simulink library "walkingRobotUtils"  (R2023a)
settings: Solver=VariableStepAuto  StartTime=0.0  StopTime=10.0  RelTol=1e-3
values from neighbouring files (symbols this model uses):
  ankle_servo_kd = 8    [robotParametersCtrl_mydiem_block_zmp.m]    (also in robotParametersCtrl_quad_modify_mydiem.m; robotParametersCtrl_quad_modify_mydiem_reaction.m)
  ankle_servo_ki = 4    [robotParametersCtrl_mydiem_block_zmp.m]    (also in robotParametersCtrl_quad_modify_mydiem.m; robotParametersCtrl_quad_modify_mydiem_reaction.m)
  ankle_servo_kp = 20    [robotParametersCtrl_mydiem_block_zmp.m]    (also in robotParametersCtrl_quad_modify_mydiem.m; robotParametersCtrl_quad_modify_mydiem_reaction.m)
  deriv_filter_coeff = 100    [robotParametersCtrl_mydiem_block_zmp.m]    (also in robotParametersCtrl_quad_modify_mydiem.m; robotParametersCtrl_quad_modify_mydiem_reaction.m)
  foot_x = 9    [robotParametersCtrl_mydiem_block_zmp.m]    (also in robotParametersCtrl_quad_modify_mydiem.m; robotParametersCtrl_quad_modify_mydiem_reaction.m)
  foot_y = 5    [robotParametersCtrl_mydiem_block_zmp.m]    (also in robotParametersCtrl_quad_modify_mydiem.m; robotParametersCtrl_quad_modify_mydiem_reaction.m)
  foot_z = 1.5    [robotParametersCtrl_mydiem_block_zmp.m]    (also in robotParametersCtrl_quad_modify_mydiem.m; robotParametersCtrl_quad_modify_mydiem_reaction.m)
  height_plane = 0.025    [robotParametersCtrl_mydiem_block_zmp.m]    (also in robotParametersCtrl_quad_modify_mydiem.m; robotParametersCtrl_quad_modify_mydiem_reaction.m)
  hip_servo_kd = 20    [robotParametersCtrl_mydiem_block_zmp.m]    (also in robotParametersCtrl_quad_modify_mydiem.m; robotParametersCtrl_quad_modify_mydiem_reaction.m)
  hip_servo_ki = 10    [robotParametersCtrl_mydiem_block_zmp.m]    (also in robotParametersCtrl_quad_modify_mydiem.m; robotParametersCtrl_quad_modify_mydiem_reaction.m)
  hip_servo_kp = 60    [robotParametersCtrl_mydiem_block_zmp.m]    (also in robotParametersCtrl_quad_modify_mydiem.m; robotParametersCtrl_quad_modify_mydiem_reaction.m)
  init_angs_L = init_angs_R    [robotParametersCtrl_mydiem_block_zmp.m]    (also in robotParametersCtrl_quad_modify_mydiem.m; robotParametersCtrl_quad_modify_mydiem_reaction.m)
  init_angs_R = [0 -sum(init_angs) init_angs(2) 0 init_angs(1)]    [robotParametersCtrl_mydiem_block_zmp.m]    (also in robotParametersCtrl_quad_modify_mydiem.m; robotParametersCtrl_quad_modify_mydiem_reaction.m)
  init_height = h +                torso_z/2 + torso_offset_z + height_plane/2    (= 39.5125)    [robotParametersCtrl_mydiem_block_zmp.m]    (also in robotParametersCtrl_quad_modify_mydiem.m; robotParametersCtrl_quad_modify_mydiem_reaction.m)
  joint_damping = 1    [robotParametersCtrl_mydiem_block_zmp.m]    (also in robotParametersCtrl_quad_modify_mydiem.m; robotParametersCtrl_quad_modify_mydiem_reaction.m)
  knee_servo_kd = 10    [robotParametersCtrl_mydiem_block_zmp.m]    (also in robotParametersCtrl_quad_modify_mydiem.m; robotParametersCtrl_quad_modify_mydiem_reaction.m)
  knee_servo_ki = 5    [robotParametersCtrl_mydiem_block_zmp.m]    (also in robotParametersCtrl_quad_modify_mydiem.m; robotParametersCtrl_quad_modify_mydiem_reaction.m)
  knee_servo_kp = 60    [robotParametersCtrl_mydiem_block_zmp.m]    (also in robotParametersCtrl_quad_modify_mydiem.m; robotParametersCtrl_quad_modify_mydiem_reaction.m)
  lower_leg_length = 20    [robotParametersCtrl_mydiem_block_zmp.m]    (also in robotParametersCtrl_quad_modify_mydiem.m; robotParametersCtrl_quad_modify_mydiem_reaction.m)
  max_torque = 20    [robotParametersCtrl_mydiem_block_zmp.m]    (also in robotParametersCtrl_quad_modify_mydiem.m; robotParametersCtrl_quad_modify_mydiem_reaction.m)
  motion_time_constant = 0.01    [robotParametersCtrl_mydiem_block_zmp.m]    (also in robotParametersCtrl_quad_modify_mydiem.m; robotParametersCtrl_quad_modify_mydiem_reaction.m)
  motor_constant = 0.02    [robotParametersCtrl_mydiem_block_zmp.m]    (also in robotParametersCtrl_quad_modify_mydiem.m; robotParametersCtrl_quad_modify_mydiem_reaction.m)
  motor_inertia = 0    [robotParametersCtrl_mydiem_block_zmp.m]    (also in robotParametersCtrl_quad_modify_mydiem.m; robotParametersCtrl_quad_modify_mydiem_reaction.m)
  motor_voltage = 24    [robotParametersCtrl_mydiem_block_zmp.m]    (also in robotParametersCtrl_quad_modify_mydiem.m; robotParametersCtrl_quad_modify_mydiem_reaction.m)
  plane_x = 25    [robotParametersCtrl_mydiem_block_zmp.m]    (also in robotParametersCtrl_quad_modify_mydiem.m; robotParametersCtrl_quad_modify_mydiem_reaction.m)
  plane_y = 3    [robotParametersCtrl_mydiem_block_zmp.m]    (also in robotParametersCtrl_quad_modify_mydiem.m; robotParametersCtrl_quad_modify_mydiem_reaction.m)
  torso_offset_x = 17    [robotParametersCtrl_mydiem_block_zmp.m]    (also in robotParametersCtrl_quad_modify_mydiem.m; robotParametersCtrl_quad_modify_mydiem_reaction.m)
  torso_offset_z = 0    [robotParametersCtrl_mydiem_block_zmp.m]    (also in robotParametersCtrl_quad_modify_mydiem.m; robotParametersCtrl_quad_modify_mydiem_reaction.m)
  torso_x = 40    [robotParametersCtrl_mydiem_block_zmp.m]    (also in robotParametersCtrl_quad_modify_mydiem.m; robotParametersCtrl_quad_modify_mydiem_reaction.m)
  torso_y = 20    [robotParametersCtrl_mydiem_block_zmp.m]    (also in robotParametersCtrl_quad_modify_mydiem.m; robotParametersCtrl_quad_modify_mydiem_reaction.m)
  torso_z = 15    [robotParametersCtrl_mydiem_block_zmp.m]    (also in robotParametersCtrl_quad_modify_mydiem.m; robotParametersCtrl_quad_modify_mydiem_reaction.m)
  upper_leg_length = 20    [robotParametersCtrl_mydiem_block_zmp.m]    (also in robotParametersCtrl_quad_modify_mydiem.m; robotParametersCtrl_quad_modify_mydiem_reaction.m)
undefined symbols (not defined in the file or in its folder): leg_width, plane_z, torso_height, torso_length, torso_offset_height, torso_offset_length, torso_width, X, Y, Z
libraries: sm_lib x110, nesl_utility x49, simulink x33, simulink_extras x32, $bdroot x28, fl_lib x7, ee_lib x3, Multibody_Multiphysics_Lib x1
(part 4 of 6)

== system walkingRobotUtils/Walking Robot (Control Design)/World and Ground ==
  Mechanism Configuration : sm_lib/Utilities/Mechanism Configuration  UniformGravity=Constant  GravityVector=[0 0 -9.80665]  GravityVectorUnits=m/s^2  LinearizationDelta=0.001  JointModeTransitionNonlinearIterations=2
  Plane Offset : sm_lib/Frames and Transforms/Rigid Transform  TranslationMethod=StandardAxis  TranslationStandardOffset=height_plane/2  TranslationStandardOffsetUnits=m  TranslationStandardAxis=-Z  TranslationCartesianOffset=[0 0 0]  TranslationCartesianOffsetUnits=m  TranslationROffset=0  TranslationROffsetUnits=m  TranslationZOffset=0  TranslationZOffsetUnits=m  TranslationThetaOffset=0  TranslationThetaOffsetUnits=deg  RotationMethod=None  RotationAngleUnits=deg  RotationStandardAxis=+Z  RotationAngle=0.0  RotationArbitraryAxis=[0 0 1]  FollAlignAxisA=+X  BaseAlignAxisA=+Y  FollAlignAxisB=+Y  BaseAlignAxisB=+Z  RotationSequenceAxes=FollowerAxes  RotationSequence=XYX  RotationSequenceAngles=[0 0 0]  RotationSequenceAnglesUnits=deg  RotationMatrix=[1 0 0; 0 1 0; 0 0 1]  Quaternion=[1 0 0 0]
  Solver Configuration : nesl_utility/Solver Configuration  PhysicalDomain=network_engine_domain  SubClassName=solver  LeftPortType=input  RightPortType=generic  Tones=[]  Harmonics=[]  SimulateNoise=off  Profile=off  UseLocalSampling=off  EnableSwitchedLinearOptims=on  FrequencyDomain=off  UseCCode=off  RelTol=0.001  AbsTol=1e-06  MinStep=1e-09  ToWorkspace=off  RevertToSquareIcSolve=off  NumHomotopyIterations=100  PhasorMode=off  PhasorModeNumHarmonics=1  ConsistencySolver=NEWTON_FTOL  IndexReductionMethod=DerivativeReplacement  DoDC=off  ResidualTolerance=1e-09  ConsistencyTolSource=GLOBAL  ConsistencyAbsTol=0.001  ConsistencyRelTol=0.001  ConsistencyTolFactor=0.001  UseLocalSolver=off  LocalSolverChoice=NE_TRAPEZOIDAL_ADVANCER  ResolveIndetEquations=on  FunctionEvalNumThread=1  LocalSolverSampleTime=0.01  DoFixedCost=off  MaxNonlinIter=3  MaxModeIter=2  ComputeImpulses=off  ImpulseIterations=2  LinearAlgebra=Sparse  LinearAlgebraNumThread=0  EquationFormulation=NE_TIME_EF  DelaysMemoryBudget=1024  AutomaticFiltering=on  FilteringTimeConstant=0.001  PartitionStorageMethod=AS_NEEDED  PartitionMemoryBudget=1024  PartitionMethod=FAST
  World Frame1 : sm_lib/Frames and Transforms/World Frame
  World Plane : sm_lib/Body Elements/Brick Solid  GraphicAmbientColor=[0.15 0.15 0.15 1.0]  BasedOnType=Density  BrickDimensions="[plane_x plane_y  height_plane]"  BrickDimensionsUnits=m  CenterOfMass=[0 0 0]  CenterOfMassUnits=m  GraphicDiffuseColor=[1.0 1.0 0.8]  Density=density  DensityUnits=kg/(m^3)  DoExposeReferenceFrame=on  GraphicEmissiveColor=[0.0 0.0 0.0 1.0]  ExportEntireGeometry=on  SerializedFrames=<Frames/>  MarkerShape=Sphere  MarkerSize=10  GraphicType=FromGeometry  InertiaType=CalculateFromGeometry  Mass=1  MassUnits=kg  MomentsOfInertia=[1 1 1]  MomentsOfInertiaUnits=kg*m^2  GraphicOpacity=0.5  ProductsOfInertia=[0 0 0]  ProductsOfInertiaUnits=kg*m^2  GraphicShininess=75  GraphicSpecularColor=[0.5 0.5 0.5 1.0]  GraphicVisPropType=SimpleVisualProperties
  W : PMIOPort  Side=Left
  G : PMIOPort  Port=2  Side=Right
  connections:
  World Frame1/RConn1 -- W/RConn1 -- Mechanism Configuration/RConn1 -- Plane Offset/LConn1 -- Solver Configuration/RConn1
  World Plane/RConn1 -- Plane Offset/RConn1
  G/RConn1 -- World Plane/LConn1

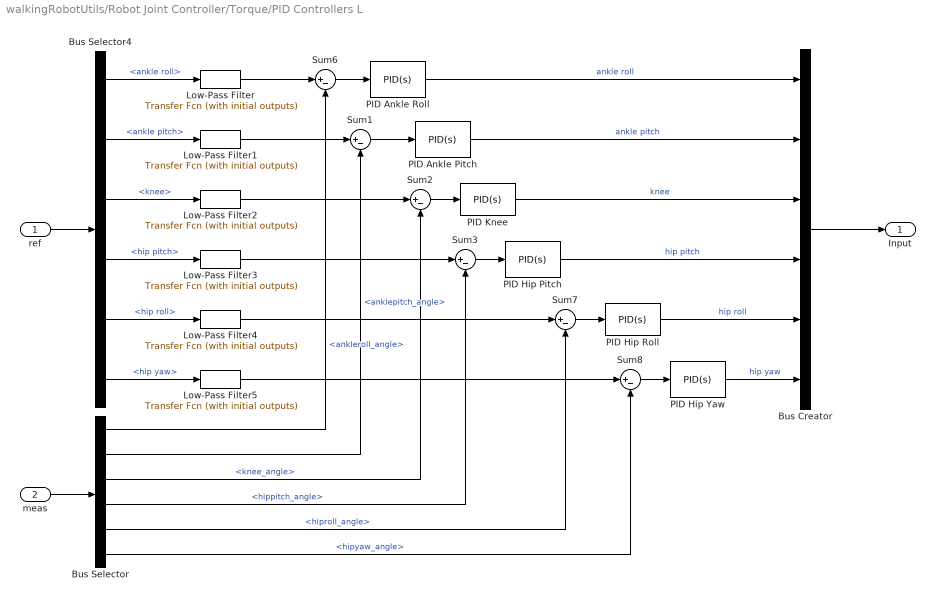
== system walkingRobotUtils/Robot Joint Controller/Torque/PID Controllers L ==
  ref : Inport
  meas : Inport  Port=2
  Bus Creator : BusCreator  Inputs=6
  Bus Selector : BusSelector  OutputSignals=ankleroll_angle,anklepitch_angle,knee_angle,hippitch_angle,hiproll_angle,hipyaw_angle
  Bus Selector4 : BusSelector  OutputSignals=ankle roll,ankle pitch,knee,hip pitch,hip roll,hip yaw
  Low-Pass Filter : simulink_extras/Additional Linear/Transfer Fcn (with initial outputs)  N=[(1/motion_time_constant)^2]  D=[1 2/motion_time_constant (1/motion_time_constant)^2]  Y0=init_angs_L(6)  U0=init_angs_L(6)
  Low-Pass Filter1 : simulink_extras/Additional Linear/Transfer Fcn (with initial outputs)  N=[(1/motion_time_constant)^2]  D=[1 2/motion_time_constant (1/motion_time_constant)^2]  Y0=init_angs_L(5)  U0=init_angs_L(5)
  Low-Pass Filter2 : simulink_extras/Additional Linear/Transfer Fcn (with initial outputs)  N=[(1/motion_time_constant)^2]  D=[1 2/motion_time_constant (1/motion_time_constant)^2]  Y0=init_angs_L(4)  U0=init_angs_L(4)
  Low-Pass Filter3 : simulink_extras/Additional Linear/Transfer Fcn (with initial outputs)  N=[(1/motion_time_constant)^2]  D=[1 2/motion_time_constant (1/motion_time_constant)^2]  Y0=init_angs_L(3)  U0=init_angs_L(3)
  Low-Pass Filter4 : simulink_extras/Additional Linear/Transfer Fcn (with initial outputs)  N=[(1/motion_time_constant)^2]  D=[1 2/motion_time_constant (1/motion_time_constant)^2]  Y0=init_angs_L(2)  U0=init_angs_L(2)
  Low-Pass Filter5 : simulink_extras/Additional Linear/Transfer Fcn (with initial outputs)  N=[(1/motion_time_constant)^2]  D=[1 2/motion_time_constant (1/motion_time_constant)^2]  Y0=init_angs_L(1)  U0=init_angs_L(1)
  PID Ankle Pitch : simulink/Continuous/PID Controller  Controller=PID  Form=Parallel  TimeDomain=Continuous-time  SampleTime=-1  IntegratorMethod=Forward Euler  FilterMethod=Forward Euler  ControllerParametersSource=internal  P=ankle_servo_kp  I=ankle_servo_ki  D=ankle_servo_kd  UseFilter=on  N=deriv_filter_coeff  TunerSelectOption=Transfer Function Based (PID Tuner App)  ZeroCross=off  InitialConditionSource=internal  InitialConditionForIntegrator=0  InitialConditionForFilter=0  DifferentiatorICPrevScaledInput=0  ExternalReset=none  TrackingMode=off  Kt=1  LimitOutput=on  UpperSaturationLimit=max_torque  LowerSaturationLimit=-max_torque  LinearizeAsGain=on  AntiWindupMode=clamping  Kb=1  POutMin=[]  POutMax=[]  IOutMin=[]  IOutMax=[]  DOutMin=[]  DOutMax=[]  NOutMin=[]  NOutMax=[]  SumOutMin=[]  SumOutMax=[]  SaturationOutMin=[]  SaturationOutMax=[]  PParamMin=[]  PParamMax=[]  IParamMin=[]  IParamMax=[]  DParamMin=[]  DParamMax=[]  NParamMin=[]  NParamMax=[]  KbParamMin=[]  KbParamMax=[]  KtParamMin=[]  KtParamMax=[]  KbOutMin=[]  KbOutMax=[]  KtOutMin=[]  KtOutMax=[]  IntegratorOutMin=[]  IntegratorOutMax=[]  FilterOutMin=[]  FilterOutMax=[]  SumI1OutMin=[]  SumI1OutMax=[]  SumI2OutMin=[]  SumI2OutMax=[]  SumI3OutMin=[]  SumI3OutMax=[]  SumI4OutMin=[]  SumI4OutMax=[]  SumDOutMin=[]  SumDOutMax=[]  DifferentiatorOutMin=[]  DifferentiatorOutMax=[]  FilterDiffOutCoefMin=[]  FilterDiffOutCoefMax=[]  ReciprocalOutMin=[]  ReciprocalOutMax=[]  SumDenOutMin=[]  SumDenOutMax=[]  SumNumOutMin=[]  SumNumOutMax=[]  DivideOutMin=[]  DivideOutMax=[]  IntegratorContinuousStateAttributes=''  IntegratorStateMustResolveToSignalObject=off  IntegratorRTWStateStorageClass=Auto  FilterContinuousStateAttributes=''  FilterStateMustResolveToSignalObject=off  FilterRTWStateStorageClass=Auto  ParallelPVariant=InternalParameters  IdealPVariant=Disabled  IVariant=InternalParameters  DVariant=InternalParameters  IntegratorVariant=Continuous  SatVariant=Enabled  AWVariant=ContClampingParallel  PCopyVariant=Disabled  TRVariant=Disabled  FdbkBlocksVariant=Forward  IdealPFdbkVariant=Disabled  SatFdbkVariant=Disabled  DerivativeFilterVariant=ContFilter  NVariant=InternalParameters  NCopyVariant=Disabled  FilterICVariant=InternalICsFilter  IntegratorICVariant=InternalICs  ExternalResetVariant=Disabled  TRSumVariant=Passthrough  SumFdbkVariant=Disabled  SumVariant=Sum_PID
  PID Ankle Roll : simulink/Continuous/PID Controller  Controller=PID  Form=Parallel  TimeDomain=Continuous-time  SampleTime=-1  IntegratorMethod=Forward Euler  FilterMethod=Forward Euler  ControllerParametersSource=internal  P=ankle_servo_kp  I=ankle_servo_ki  D=ankle_servo_kd  UseFilter=on  N=deriv_filter_coeff  TunerSelectOption=Transfer Function Based (PID Tuner App)  ZeroCross=off  InitialConditionSource=internal  InitialConditionForIntegrator=0  InitialConditionForFilter=0  DifferentiatorICPrevScaledInput=0  ExternalReset=none  TrackingMode=off  Kt=1  LimitOutput=on  UpperSaturationLimit=max_torque  LowerSaturationLimit=-max_torque  LinearizeAsGain=on  AntiWindupMode=clamping  Kb=1  POutMin=[]  POutMax=[]  IOutMin=[]  IOutMax=[]  DOutMin=[]  DOutMax=[]  NOutMin=[]  NOutMax=[]  SumOutMin=[]  SumOutMax=[]  SaturationOutMin=[]  SaturationOutMax=[]  PParamMin=[]  PParamMax=[]  IParamMin=[]  IParamMax=[]  DParamMin=[]  DParamMax=[]  NParamMin=[]  NParamMax=[]  KbParamMin=[]  KbParamMax=[]  KtParamMin=[]  KtParamMax=[]  KbOutMin=[]  KbOutMax=[]  KtOutMin=[]  KtOutMax=[]  IntegratorOutMin=[]  IntegratorOutMax=[]  FilterOutMin=[]  FilterOutMax=[]  SumI1OutMin=[]  SumI1OutMax=[]  SumI2OutMin=[]  SumI2OutMax=[]  SumI3OutMin=[]  SumI3OutMax=[]  SumI4OutMin=[]  SumI4OutMax=[]  SumDOutMin=[]  SumDOutMax=[]  DifferentiatorOutMin=[]  DifferentiatorOutMax=[]  FilterDiffOutCoefMin=[]  FilterDiffOutCoefMax=[]  ReciprocalOutMin=[]  ReciprocalOutMax=[]  SumDenOutMin=[]  SumDenOutMax=[]  SumNumOutMin=[]  SumNumOutMax=[]  DivideOutMin=[]  DivideOutMax=[]  IntegratorContinuousStateAttributes=''  IntegratorStateMustResolveToSignalObject=off  IntegratorRTWStateStorageClass=Auto  FilterContinuousStateAttributes=''  FilterStateMustResolveToSignalObject=off  FilterRTWStateStorageClass=Auto  ParallelPVariant=InternalParameters  IdealPVariant=Disabled  IVariant=InternalParameters  DVariant=InternalParameters  IntegratorVariant=Continuous  SatVariant=Enabled  AWVariant=ContClampingParallel  PCopyVariant=Disabled  TRVariant=Disabled  FdbkBlocksVariant=Forward  IdealPFdbkVariant=Disabled  SatFdbkVariant=Disabled  DerivativeFilterVariant=ContFilter  NVariant=InternalParameters  NCopyVariant=Disabled  FilterICVariant=InternalICsFilter  IntegratorICVariant=InternalICs  ExternalResetVariant=Disabled  TRSumVariant=Passthrough  SumFdbkVariant=Disabled  SumVariant=Sum_PID
  PID Hip Pitch : simulink/Continuous/PID Controller  Controller=PID  Form=Parallel  TimeDomain=Continuous-time  SampleTime=-1  IntegratorMethod=Forward Euler  FilterMethod=Forward Euler  ControllerParametersSource=internal  P=hip_servo_kp  I=hip_servo_ki  D=hip_servo_kd  UseFilter=on  N=deriv_filter_coeff  TunerSelectOption=Transfer Function Based (PID Tuner App)  ZeroCross=off  InitialConditionSource=internal  InitialConditionForIntegrator=0  InitialConditionForFilter=0  DifferentiatorICPrevScaledInput=0  ExternalReset=none  TrackingMode=off  Kt=1  LimitOutput=on  UpperSaturationLimit=max_torque  LowerSaturationLimit=-max_torque  LinearizeAsGain=on  AntiWindupMode=clamping  Kb=1  POutMin=[]  POutMax=[]  IOutMin=[]  IOutMax=[]  DOutMin=[]  DOutMax=[]  NOutMin=[]  NOutMax=[]  SumOutMin=[]  SumOutMax=[]  SaturationOutMin=[]  SaturationOutMax=[]  PParamMin=[]  PParamMax=[]  IParamMin=[]  IParamMax=[]  DParamMin=[]  DParamMax=[]  NParamMin=[]  NParamMax=[]  KbParamMin=[]  KbParamMax=[]  KtParamMin=[]  KtParamMax=[]  KbOutMin=[]  KbOutMax=[]  KtOutMin=[]  KtOutMax=[]  IntegratorOutMin=[]  IntegratorOutMax=[]  FilterOutMin=[]  FilterOutMax=[]  SumI1OutMin=[]  SumI1OutMax=[]  SumI2OutMin=[]  SumI2OutMax=[]  SumI3OutMin=[]  SumI3OutMax=[]  SumI4OutMin=[]  SumI4OutMax=[]  SumDOutMin=[]  SumDOutMax=[]  DifferentiatorOutMin=[]  DifferentiatorOutMax=[]  FilterDiffOutCoefMin=[]  FilterDiffOutCoefMax=[]  ReciprocalOutMin=[]  ReciprocalOutMax=[]  SumDenOutMin=[]  SumDenOutMax=[]  SumNumOutMin=[]  SumNumOutMax=[]  DivideOutMin=[]  DivideOutMax=[]  IntegratorContinuousStateAttributes=''  IntegratorStateMustResolveToSignalObject=off  IntegratorRTWStateStorageClass=Auto  FilterContinuousStateAttributes=''  FilterStateMustResolveToSignalObject=off  FilterRTWStateStorageClass=Auto  ParallelPVariant=InternalParameters  IdealPVariant=Disabled  IVariant=InternalParameters  DVariant=InternalParameters  IntegratorVariant=Continuous  SatVariant=Enabled  AWVariant=ContClampingParallel  PCopyVariant=Disabled  TRVariant=Disabled  FdbkBlocksVariant=Forward  IdealPFdbkVariant=Disabled  SatFdbkVariant=Disabled  DerivativeFilterVariant=ContFilter  NVariant=InternalParameters  NCopyVariant=Disabled  FilterICVariant=InternalICsFilter  IntegratorICVariant=InternalICs  ExternalResetVariant=Disabled  TRSumVariant=Passthrough  SumFdbkVariant=Disabled  SumVariant=Sum_PID
  PID Hip Roll : simulink/Continuous/PID Controller  Controller=PID  Form=Parallel  TimeDomain=Continuous-time  SampleTime=-1  IntegratorMethod=Forward Euler  FilterMethod=Forward Euler  ControllerParametersSource=internal  P=hip_servo_kp  I=hip_servo_ki  D=hip_servo_kd  UseFilter=on  N=deriv_filter_coeff  TunerSelectOption=Transfer Function Based (PID Tuner App)  ZeroCross=off  InitialConditionSource=internal  InitialConditionForIntegrator=0  InitialConditionForFilter=0  DifferentiatorICPrevScaledInput=0  ExternalReset=none  TrackingMode=off  Kt=1  LimitOutput=on  UpperSaturationLimit=max_torque  LowerSaturationLimit=-max_torque  LinearizeAsGain=on  AntiWindupMode=clamping  Kb=1  POutMin=[]  POutMax=[]  IOutMin=[]  IOutMax=[]  DOutMin=[]  DOutMax=[]  NOutMin=[]  NOutMax=[]  SumOutMin=[]  SumOutMax=[]  SaturationOutMin=[]  SaturationOutMax=[]  PParamMin=[]  PParamMax=[]  IParamMin=[]  IParamMax=[]  DParamMin=[]  DParamMax=[]  NParamMin=[]  NParamMax=[]  KbParamMin=[]  KbParamMax=[]  KtParamMin=[]  KtParamMax=[]  KbOutMin=[]  KbOutMax=[]  KtOutMin=[]  KtOutMax=[]  IntegratorOutMin=[]  IntegratorOutMax=[]  FilterOutMin=[]  FilterOutMax=[]  SumI1OutMin=[]  SumI1OutMax=[]  SumI2OutMin=[]  SumI2OutMax=[]  SumI3OutMin=[]  SumI3OutMax=[]  SumI4OutMin=[]  SumI4OutMax=[]  SumDOutMin=[]  SumDOutMax=[]  DifferentiatorOutMin=[]  DifferentiatorOutMax=[]  FilterDiffOutCoefMin=[]  FilterDiffOutCoefMax=[]  ReciprocalOutMin=[]  ReciprocalOutMax=[]  SumDenOutMin=[]  SumDenOutMax=[]  SumNumOutMin=[]  SumNumOutMax=[]  DivideOutMin=[]  DivideOutMax=[]  IntegratorContinuousStateAttributes=''  IntegratorStateMustResolveToSignalObject=off  IntegratorRTWStateStorageClass=Auto  FilterContinuousStateAttributes=''  FilterStateMustResolveToSignalObject=off  FilterRTWStateStorageClass=Auto  ParallelPVariant=InternalParameters  IdealPVariant=Disabled  IVariant=InternalParameters  DVariant=InternalParameters  IntegratorVariant=Continuous  SatVariant=Enabled  AWVariant=ContClampingParallel  PCopyVariant=Disabled  TRVariant=Disabled  FdbkBlocksVariant=Forward  IdealPFdbkVariant=Disabled  SatFdbkVariant=Disabled  DerivativeFilterVariant=ContFilter  NVariant=InternalParameters  NCopyVariant=Disabled  FilterICVariant=InternalICsFilter  IntegratorICVariant=InternalICs  ExternalResetVariant=Disabled  TRSumVariant=Passthrough  SumFdbkVariant=Disabled  SumVariant=Sum_PID
  PID Hip Yaw : simulink/Continuous/PID Controller  Controller=PID  Form=Parallel  TimeDomain=Continuous-time  SampleTime=-1  IntegratorMethod=Forward Euler  FilterMethod=Forward Euler  ControllerParametersSource=internal  P=hip_servo_kp  I=hip_servo_ki  D=hip_servo_kd  UseFilter=on  N=deriv_filter_coeff  TunerSelectOption=Transfer Function Based (PID Tuner App)  ZeroCross=off  InitialConditionSource=internal  InitialConditionForIntegrator=0  InitialConditionForFilter=0  DifferentiatorICPrevScaledInput=0  ExternalReset=none  TrackingMode=off  Kt=1  LimitOutput=on  UpperSaturationLimit=max_torque  LowerSaturationLimit=-max_torque  LinearizeAsGain=on  AntiWindupMode=clamping  Kb=1  POutMin=[]  POutMax=[]  IOutMin=[]  IOutMax=[]  DOutMin=[]  DOutMax=[]  NOutMin=[]  NOutMax=[]  SumOutMin=[]  SumOutMax=[]  SaturationOutMin=[]  SaturationOutMax=[]  PParamMin=[]  PParamMax=[]  IParamMin=[]  IParamMax=[]  DParamMin=[]  DParamMax=[]  NParamMin=[]  NParamMax=[]  KbParamMin=[]  KbParamMax=[]  KtParamMin=[]  KtParamMax=[]  KbOutMin=[]  KbOutMax=[]  KtOutMin=[]  KtOutMax=[]  IntegratorOutMin=[]  IntegratorOutMax=[]  FilterOutMin=[]  FilterOutMax=[]  SumI1OutMin=[]  SumI1OutMax=[]  SumI2OutMin=[]  SumI2OutMax=[]  SumI3OutMin=[]  SumI3OutMax=[]  SumI4OutMin=[]  SumI4OutMax=[]  SumDOutMin=[]  SumDOutMax=[]  DifferentiatorOutMin=[]  DifferentiatorOutMax=[]  FilterDiffOutCoefMin=[]  FilterDiffOutCoefMax=[]  ReciprocalOutMin=[]  ReciprocalOutMax=[]  SumDenOutMin=[]  SumDenOutMax=[]  SumNumOutMin=[]  SumNumOutMax=[]  DivideOutMin=[]  DivideOutMax=[]  IntegratorContinuousStateAttributes=''  IntegratorStateMustResolveToSignalObject=off  IntegratorRTWStateStorageClass=Auto  FilterContinuousStateAttributes=''  FilterStateMustResolveToSignalObject=off  FilterRTWStateStorageClass=Auto  ParallelPVariant=InternalParameters  IdealPVariant=Disabled  IVariant=InternalParameters  DVariant=InternalParameters  IntegratorVariant=Continuous  SatVariant=Enabled  AWVariant=ContClampingParallel  PCopyVariant=Disabled  TRVariant=Disabled  FdbkBlocksVariant=Forward  IdealPFdbkVariant=Disabled  SatFdbkVariant=Disabled  DerivativeFilterVariant=ContFilter  NVariant=InternalParameters  NCopyVariant=Disabled  FilterICVariant=InternalICsFilter  IntegratorICVariant=InternalICs  ExternalResetVariant=Disabled  TRSumVariant=Passthrough  SumFdbkVariant=Disabled  SumVariant=Sum_PID
  PID Knee : simulink/Continuous/PID Controller  Controller=PID  Form=Parallel  TimeDomain=Continuous-time  SampleTime=-1  IntegratorMethod=Forward Euler  FilterMethod=Forward Euler  ControllerParametersSource=internal  P=knee_servo_kp  I=knee_servo_ki  D=knee_servo_kd  UseFilter=on  N=deriv_filter_coeff  TunerSelectOption=Transfer Function Based (PID Tuner App)  ZeroCross=off  InitialConditionSource=internal  InitialConditionForIntegrator=0  InitialConditionForFilter=0  DifferentiatorICPrevScaledInput=0  ExternalReset=none  TrackingMode=off  Kt=1  LimitOutput=on  UpperSaturationLimit=max_torque  LowerSaturationLimit=-max_torque  LinearizeAsGain=on  AntiWindupMode=clamping  Kb=1  POutMin=[]  POutMax=[]  IOutMin=[]  IOutMax=[]  DOutMin=[]  DOutMax=[]  NOutMin=[]  NOutMax=[]  SumOutMin=[]  SumOutMax=[]  SaturationOutMin=[]  SaturationOutMax=[]  PParamMin=[]  PParamMax=[]  IParamMin=[]  IParamMax=[]  DParamMin=[]  DParamMax=[]  NParamMin=[]  NParamMax=[]  KbParamMin=[]  KbParamMax=[]  KtParamMin=[]  KtParamMax=[]  KbOutMin=[]  KbOutMax=[]  KtOutMin=[]  KtOutMax=[]  IntegratorOutMin=[]  IntegratorOutMax=[]  FilterOutMin=[]  FilterOutMax=[]  SumI1OutMin=[]  SumI1OutMax=[]  SumI2OutMin=[]  SumI2OutMax=[]  SumI3OutMin=[]  SumI3OutMax=[]  SumI4OutMin=[]  SumI4OutMax=[]  SumDOutMin=[]  SumDOutMax=[]  DifferentiatorOutMin=[]  DifferentiatorOutMax=[]  FilterDiffOutCoefMin=[]  FilterDiffOutCoefMax=[]  ReciprocalOutMin=[]  ReciprocalOutMax=[]  SumDenOutMin=[]  SumDenOutMax=[]  SumNumOutMin=[]  SumNumOutMax=[]  DivideOutMin=[]  DivideOutMax=[]  IntegratorContinuousStateAttributes=''  IntegratorStateMustResolveToSignalObject=off  IntegratorRTWStateStorageClass=Auto  FilterContinuousStateAttributes=''  FilterStateMustResolveToSignalObject=off  FilterRTWStateStorageClass=Auto  ParallelPVariant=InternalParameters  IdealPVariant=Disabled  IVariant=InternalParameters  DVariant=InternalParameters  IntegratorVariant=Continuous  SatVariant=Enabled  AWVariant=ContClampingParallel  PCopyVariant=Disabled  TRVariant=Disabled  FdbkBlocksVariant=Forward  IdealPFdbkVariant=Disabled  SatFdbkVariant=Disabled  DerivativeFilterVariant=ContFilter  NVariant=InternalParameters  NCopyVariant=Disabled  FilterICVariant=InternalICsFilter  IntegratorICVariant=InternalICs  ExternalResetVariant=Disabled  TRSumVariant=Passthrough  SumFdbkVariant=Disabled  SumVariant=Sum_PID
  Sum{1..3,6..8} (6 alike) : Sum  Inputs=|+-
  Input : Outport  VectorParamsAs1DForOutWhenUnconnected=off
  wires:
  meas/1 -> Bus Selector/1
  Bus Selector/2 -> Sum1/2  "<anklepitch_angle>"
  Bus Selector/4 -> Sum3/2  "<hippitch_angle>"
  Low-Pass Filter4/1 -> Sum7/1
  Low-Pass Filter2/1 -> Sum2/1
  Sum8/1 -> PID Hip Yaw/1
  Bus Selector/1 -> Sum6/2  "<ankleroll_angle>"
  Bus Creator/1 -> Input/1
  Low-Pass Filter1/1 -> Sum1/1
  Bus Selector/5 -> Sum7/2  "<hiproll_angle>"
  PID Hip Pitch/1 -> Bus Creator/4  "hip pitch"
  Bus Selector/6 -> Sum8/2  "<hipyaw_angle>"
  Low-Pass Filter3/1 -> Sum3/1
  PID Ankle Roll/1 -> Bus Creator/1  "ankle roll"
  Sum1/1 -> PID Ankle Pitch/1
  Sum2/1 -> PID Knee/1
  ref/1 -> Bus Selector4/1
  Sum3/1 -> PID Hip Pitch/1
  Bus Selector4/5 -> Low-Pass Filter4/1  "<hip roll>"
  Sum7/1 -> PID Hip Roll/1
  Bus Selector/3 -> Sum2/2  "<knee_angle>"
  Sum6/1 -> PID Ankle Roll/1
  Bus Selector4/1 -> Low-Pass Filter/1  "<ankle roll>"
  Bus Selector4/3 -> Low-Pass Filter2/1  "<knee>"
  PID Knee/1 -> Bus Creator/3  "knee"
  PID Hip Yaw/1 -> Bus Creator/6  "hip yaw"
  PID Ankle Pitch/1 -> Bus Creator/2  "ankle pitch"
  Bus Selector4/4 -> Low-Pass Filter3/1  "<hip pitch>"
  Bus Selector4/2 -> Low-Pass Filter1/1  "<ankle pitch>"
  PID Hip Roll/1 -> Bus Creator/5  "hip roll"
  Bus Selector4/6 -> Low-Pass Filter5/1  "<hip yaw>"
  Low-Pass Filter/1 -> Sum6/1
  Low-Pass Filter5/1 -> Sum8/1

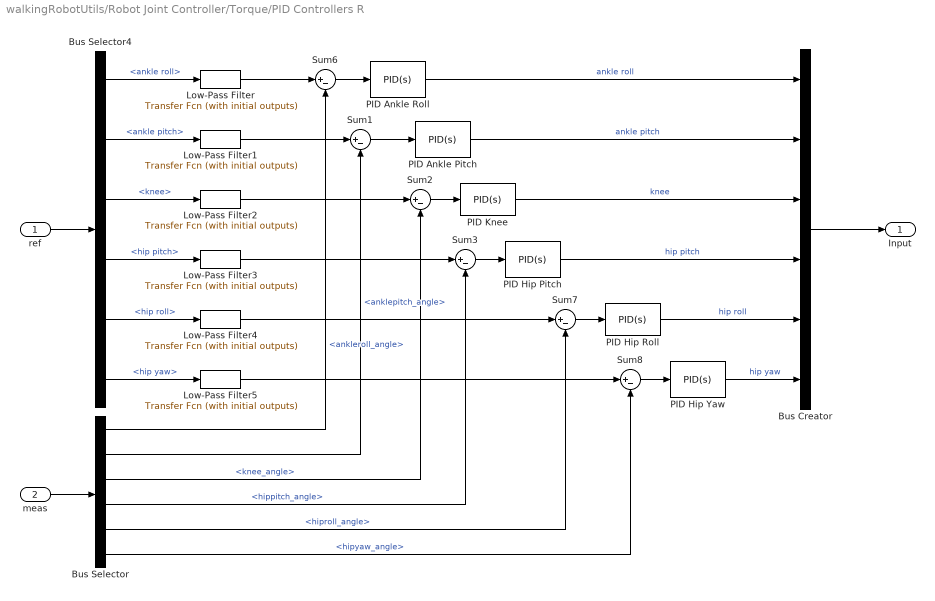
== system walkingRobotUtils/Robot Joint Controller/Torque/PID Controllers R ==
  ref : Inport
  meas : Inport  Port=2
  Bus Creator : BusCreator  Inputs=6
  Bus Selector : BusSelector  OutputSignals=ankleroll_angle,anklepitch_angle,knee_angle,hippitch_angle,hiproll_angle,hipyaw_angle
  Bus Selector4 : BusSelector  OutputSignals=ankle roll,ankle pitch,knee,hip pitch,hip roll,hip yaw
  Low-Pass Filter : simulink_extras/Additional Linear/Transfer Fcn (with initial outputs)  N=[(1/motion_time_constant)^2]  D=[1 2/motion_time_constant (1/motion_time_constant)^2]  Y0=init_angs_R(6)  U0=init_angs_R(6)
  Low-Pass Filter1 : simulink_extras/Additional Linear/Transfer Fcn (with initial outputs)  N=[(1/motion_time_constant)^2]  D=[1 2/motion_time_constant (1/motion_time_constant)^2]  Y0=init_angs_R(5)  U0=init_angs_R(5)
  Low-Pass Filter2 : simulink_extras/Additional Linear/Transfer Fcn (with initial outputs)  N=[(1/motion_time_constant)^2]  D=[1 2/motion_time_constant (1/motion_time_constant)^2]  Y0=init_angs_R(4)  U0=init_angs_R(4)
  Low-Pass Filter3 : simulink_extras/Additional Linear/Transfer Fcn (with initial outputs)  N=[(1/motion_time_constant)^2]  D=[1 2/motion_time_constant (1/motion_time_constant)^2]  Y0=init_angs_R(3)  U0=init_angs_R(3)
  Low-Pass Filter4 : simulink_extras/Additional Linear/Transfer Fcn (with initial outputs)  N=[(1/motion_time_constant)^2]  D=[1 2/motion_time_constant (1/motion_time_constant)^2]  Y0=init_angs_R(2)  U0=init_angs_R(2)
  Low-Pass Filter5 : simulink_extras/Additional Linear/Transfer Fcn (with initial outputs)  N=[(1/motion_time_constant)^2]  D=[1 2/motion_time_constant (1/motion_time_constant)^2]  Y0=init_angs_R(1)  U0=init_angs_R(1)
  PID Ankle Pitch : simulink/Continuous/PID Controller  Controller=PID  Form=Parallel  TimeDomain=Continuous-time  SampleTime=-1  IntegratorMethod=Forward Euler  FilterMethod=Forward Euler  ControllerParametersSource=internal  P=ankle_servo_kp  I=ankle_servo_ki  D=ankle_servo_kd  UseFilter=on  N=deriv_filter_coeff  TunerSelectOption=Transfer Function Based (PID Tuner App)  ZeroCross=off  InitialConditionSource=internal  InitialConditionForIntegrator=0  InitialConditionForFilter=0  DifferentiatorICPrevScaledInput=0  ExternalReset=none  TrackingMode=off  Kt=1  LimitOutput=on  UpperSaturationLimit=max_torque  LowerSaturationLimit=-max_torque  LinearizeAsGain=on  AntiWindupMode=clamping  Kb=1  POutMin=[]  POutMax=[]  IOutMin=[]  IOutMax=[]  DOutMin=[]  DOutMax=[]  NOutMin=[]  NOutMax=[]  SumOutMin=[]  SumOutMax=[]  SaturationOutMin=[]  SaturationOutMax=[]  PParamMin=[]  PParamMax=[]  IParamMin=[]  IParamMax=[]  DParamMin=[]  DParamMax=[]  NParamMin=[]  NParamMax=[]  KbParamMin=[]  KbParamMax=[]  KtParamMin=[]  KtParamMax=[]  KbOutMin=[]  KbOutMax=[]  KtOutMin=[]  KtOutMax=[]  IntegratorOutMin=[]  IntegratorOutMax=[]  FilterOutMin=[]  FilterOutMax=[]  SumI1OutMin=[]  SumI1OutMax=[]  SumI2OutMin=[]  SumI2OutMax=[]  SumI3OutMin=[]  SumI3OutMax=[]  SumI4OutMin=[]  SumI4OutMax=[]  SumDOutMin=[]  SumDOutMax=[]  DifferentiatorOutMin=[]  DifferentiatorOutMax=[]  FilterDiffOutCoefMin=[]  FilterDiffOutCoefMax=[]  ReciprocalOutMin=[]  ReciprocalOutMax=[]  SumDenOutMin=[]  SumDenOutMax=[]  SumNumOutMin=[]  SumNumOutMax=[]  DivideOutMin=[]  DivideOutMax=[]  IntegratorContinuousStateAttributes=''  IntegratorStateMustResolveToSignalObject=off  IntegratorRTWStateStorageClass=Auto  FilterContinuousStateAttributes=''  FilterStateMustResolveToSignalObject=off  FilterRTWStateStorageClass=Auto  ParallelPVariant=InternalParameters  IdealPVariant=Disabled  IVariant=InternalParameters  DVariant=InternalParameters  IntegratorVariant=Continuous  SatVariant=Enabled  AWVariant=ContClampingParallel  PCopyVariant=Disabled  TRVariant=Disabled  FdbkBlocksVariant=Forward  IdealPFdbkVariant=Disabled  SatFdbkVariant=Disabled  DerivativeFilterVariant=ContFilter  NVariant=InternalParameters  NCopyVariant=Disabled  FilterICVariant=InternalICsFilter  IntegratorICVariant=InternalICs  ExternalResetVariant=Disabled  TRSumVariant=Passthrough  SumFdbkVariant=Disabled  SumVariant=Sum_PID
  PID Ankle Roll : simulink/Continuous/PID Controller  Controller=PID  Form=Parallel  TimeDomain=Continuous-time  SampleTime=-1  IntegratorMethod=Forward Euler  FilterMethod=Forward Euler  ControllerParametersSource=internal  P=ankle_servo_kp  I=ankle_servo_ki  D=ankle_servo_kd  UseFilter=on  N=deriv_filter_coeff  TunerSelectOption=Transfer Function Based (PID Tuner App)  ZeroCross=off  InitialConditionSource=internal  InitialConditionForIntegrator=0  InitialConditionForFilter=0  DifferentiatorICPrevScaledInput=0  ExternalReset=none  TrackingMode=off  Kt=1  LimitOutput=on  UpperSaturationLimit=max_torque  LowerSaturationLimit=-max_torque  LinearizeAsGain=on  AntiWindupMode=clamping  Kb=1  POutMin=[]  POutMax=[]  IOutMin=[]  IOutMax=[]  DOutMin=[]  DOutMax=[]  NOutMin=[]  NOutMax=[]  SumOutMin=[]  SumOutMax=[]  SaturationOutMin=[]  SaturationOutMax=[]  PParamMin=[]  PParamMax=[]  IParamMin=[]  IParamMax=[]  DParamMin=[]  DParamMax=[]  NParamMin=[]  NParamMax=[]  KbParamMin=[]  KbParamMax=[]  KtParamMin=[]  KtParamMax=[]  KbOutMin=[]  KbOutMax=[]  KtOutMin=[]  KtOutMax=[]  IntegratorOutMin=[]  IntegratorOutMax=[]  FilterOutMin=[]  FilterOutMax=[]  SumI1OutMin=[]  SumI1OutMax=[]  SumI2OutMin=[]  SumI2OutMax=[]  SumI3OutMin=[]  SumI3OutMax=[]  SumI4OutMin=[]  SumI4OutMax=[]  SumDOutMin=[]  SumDOutMax=[]  DifferentiatorOutMin=[]  DifferentiatorOutMax=[]  FilterDiffOutCoefMin=[]  FilterDiffOutCoefMax=[]  ReciprocalOutMin=[]  ReciprocalOutMax=[]  SumDenOutMin=[]  SumDenOutMax=[]  SumNumOutMin=[]  SumNumOutMax=[]  DivideOutMin=[]  DivideOutMax=[]  IntegratorContinuousStateAttributes=''  IntegratorStateMustResolveToSignalObject=off  IntegratorRTWStateStorageClass=Auto  FilterContinuousStateAttributes=''  FilterStateMustResolveToSignalObject=off  FilterRTWStateStorageClass=Auto  ParallelPVariant=InternalParameters  IdealPVariant=Disabled  IVariant=InternalParameters  DVariant=InternalParameters  IntegratorVariant=Continuous  SatVariant=Enabled  AWVariant=ContClampingParallel  PCopyVariant=Disabled  TRVariant=Disabled  FdbkBlocksVariant=Forward  IdealPFdbkVariant=Disabled  SatFdbkVariant=Disabled  DerivativeFilterVariant=ContFilter  NVariant=InternalParameters  NCopyVariant=Disabled  FilterICVariant=InternalICsFilter  IntegratorICVariant=InternalICs  ExternalResetVariant=Disabled  TRSumVariant=Passthrough  SumFdbkVariant=Disabled  SumVariant=Sum_PID
  PID Hip Pitch : simulink/Continuous/PID Controller  Controller=PID  Form=Parallel  TimeDomain=Continuous-time  SampleTime=-1  IntegratorMethod=Forward Euler  FilterMethod=Forward Euler  ControllerParametersSource=internal  P=hip_servo_kp  I=hip_servo_ki  D=hip_servo_kd  UseFilter=on  N=deriv_filter_coeff  TunerSelectOption=Transfer Function Based (PID Tuner App)  ZeroCross=off  InitialConditionSource=internal  InitialConditionForIntegrator=0  InitialConditionForFilter=0  DifferentiatorICPrevScaledInput=0  ExternalReset=none  TrackingMode=off  Kt=1  LimitOutput=on  UpperSaturationLimit=max_torque  LowerSaturationLimit=-max_torque  LinearizeAsGain=on  AntiWindupMode=clamping  Kb=1  POutMin=[]  POutMax=[]  IOutMin=[]  IOutMax=[]  DOutMin=[]  DOutMax=[]  NOutMin=[]  NOutMax=[]  SumOutMin=[]  SumOutMax=[]  SaturationOutMin=[]  SaturationOutMax=[]  PParamMin=[]  PParamMax=[]  IParamMin=[]  IParamMax=[]  DParamMin=[]  DParamMax=[]  NParamMin=[]  NParamMax=[]  KbParamMin=[]  KbParamMax=[]  KtParamMin=[]  KtParamMax=[]  KbOutMin=[]  KbOutMax=[]  KtOutMin=[]  KtOutMax=[]  IntegratorOutMin=[]  IntegratorOutMax=[]  FilterOutMin=[]  FilterOutMax=[]  SumI1OutMin=[]  SumI1OutMax=[]  SumI2OutMin=[]  SumI2OutMax=[]  SumI3OutMin=[]  SumI3OutMax=[]  SumI4OutMin=[]  SumI4OutMax=[]  SumDOutMin=[]  SumDOutMax=[]  DifferentiatorOutMin=[]  DifferentiatorOutMax=[]  FilterDiffOutCoefMin=[]  FilterDiffOutCoefMax=[]  ReciprocalOutMin=[]  ReciprocalOutMax=[]  SumDenOutMin=[]  SumDenOutMax=[]  SumNumOutMin=[]  SumNumOutMax=[]  DivideOutMin=[]  DivideOutMax=[]  IntegratorContinuousStateAttributes=''  IntegratorStateMustResolveToSignalObject=off  IntegratorRTWStateStorageClass=Auto  FilterContinuousStateAttributes=''  FilterStateMustResolveToSignalObject=off  FilterRTWStateStorageClass=Auto  ParallelPVariant=InternalParameters  IdealPVariant=Disabled  IVariant=InternalParameters  DVariant=InternalParameters  IntegratorVariant=Continuous  SatVariant=Enabled  AWVariant=ContClampingParallel  PCopyVariant=Disabled  TRVariant=Disabled  FdbkBlocksVariant=Forward  IdealPFdbkVariant=Disabled  SatFdbkVariant=Disabled  DerivativeFilterVariant=ContFilter  NVariant=InternalParameters  NCopyVariant=Disabled  FilterICVariant=InternalICsFilter  IntegratorICVariant=InternalICs  ExternalResetVariant=Disabled  TRSumVariant=Passthrough  SumFdbkVariant=Disabled  SumVariant=Sum_PID
  PID Hip Roll : simulink/Continuous/PID Controller  Controller=PID  Form=Parallel  TimeDomain=Continuous-time  SampleTime=-1  IntegratorMethod=Forward Euler  FilterMethod=Forward Euler  ControllerParametersSource=internal  P=hip_servo_kp  I=hip_servo_ki  D=hip_servo_kd  UseFilter=on  N=deriv_filter_coeff  TunerSelectOption=Transfer Function Based (PID Tuner App)  ZeroCross=off  InitialConditionSource=internal  InitialConditionForIntegrator=0  InitialConditionForFilter=0  DifferentiatorICPrevScaledInput=0  ExternalReset=none  TrackingMode=off  Kt=1  LimitOutput=on  UpperSaturationLimit=max_torque  LowerSaturationLimit=-max_torque  LinearizeAsGain=on  AntiWindupMode=clamping  Kb=1  POutMin=[]  POutMax=[]  IOutMin=[]  IOutMax=[]  DOutMin=[]  DOutMax=[]  NOutMin=[]  NOutMax=[]  SumOutMin=[]  SumOutMax=[]  SaturationOutMin=[]  SaturationOutMax=[]  PParamMin=[]  PParamMax=[]  IParamMin=[]  IParamMax=[]  DParamMin=[]  DParamMax=[]  NParamMin=[]  NParamMax=[]  KbParamMin=[]  KbParamMax=[]  KtParamMin=[]  KtParamMax=[]  KbOutMin=[]  KbOutMax=[]  KtOutMin=[]  KtOutMax=[]  IntegratorOutMin=[]  IntegratorOutMax=[]  FilterOutMin=[]  FilterOutMax=[]  SumI1OutMin=[]  SumI1OutMax=[]  SumI2OutMin=[]  SumI2OutMax=[]  SumI3OutMin=[]  SumI3OutMax=[]  SumI4OutMin=[]  SumI4OutMax=[]  SumDOutMin=[]  SumDOutMax=[]  DifferentiatorOutMin=[]  DifferentiatorOutMax=[]  FilterDiffOutCoefMin=[]  FilterDiffOutCoefMax=[]  ReciprocalOutMin=[]  ReciprocalOutMax=[]  SumDenOutMin=[]  SumDenOutMax=[]  SumNumOutMin=[]  SumNumOutMax=[]  DivideOutMin=[]  DivideOutMax=[]  IntegratorContinuousStateAttributes=''  IntegratorStateMustResolveToSignalObject=off  IntegratorRTWStateStorageClass=Auto  FilterContinuousStateAttributes=''  FilterStateMustResolveToSignalObject=off  FilterRTWStateStorageClass=Auto  ParallelPVariant=InternalParameters  IdealPVariant=Disabled  IVariant=InternalParameters  DVariant=InternalParameters  IntegratorVariant=Continuous  SatVariant=Enabled  AWVariant=ContClampingParallel  PCopyVariant=Disabled  TRVariant=Disabled  FdbkBlocksVariant=Forward  IdealPFdbkVariant=Disabled  SatFdbkVariant=Disabled  DerivativeFilterVariant=ContFilter  NVariant=InternalParameters  NCopyVariant=Disabled  FilterICVariant=InternalICsFilter  IntegratorICVariant=InternalICs  ExternalResetVariant=Disabled  TRSumVariant=Passthrough  SumFdbkVariant=Disabled  SumVariant=Sum_PID
  PID Hip Yaw : simulink/Continuous/PID Controller  Controller=PID  Form=Parallel  TimeDomain=Continuous-time  SampleTime=-1  IntegratorMethod=Forward Euler  FilterMethod=Forward Euler  ControllerParametersSource=internal  P=hip_servo_kp  I=hip_servo_ki  D=hip_servo_kd  UseFilter=on  N=deriv_filter_coeff  TunerSelectOption=Transfer Function Based (PID Tuner App)  ZeroCross=off  InitialConditionSource=internal  InitialConditionForIntegrator=0  InitialConditionForFilter=0  DifferentiatorICPrevScaledInput=0  ExternalReset=none  TrackingMode=off  Kt=1  LimitOutput=on  UpperSaturationLimit=max_torque  LowerSaturationLimit=-max_torque  LinearizeAsGain=on  AntiWindupMode=clamping  Kb=1  POutMin=[]  POutMax=[]  IOutMin=[]  IOutMax=[]  DOutMin=[]  DOutMax=[]  NOutMin=[]  NOutMax=[]  SumOutMin=[]  SumOutMax=[]  SaturationOutMin=[]  SaturationOutMax=[]  PParamMin=[]  PParamMax=[]  IParamMin=[]  IParamMax=[]  DParamMin=[]  DParamMax=[]  NParamMin=[]  NParamMax=[]  KbParamMin=[]  KbParamMax=[]  KtParamMin=[]  KtParamMax=[]  KbOutMin=[]  KbOutMax=[]  KtOutMin=[]  KtOutMax=[]  IntegratorOutMin=[]  IntegratorOutMax=[]  FilterOutMin=[]  FilterOutMax=[]  SumI1OutMin=[]  SumI1OutMax=[]  SumI2OutMin=[]  SumI2OutMax=[]  SumI3OutMin=[]  SumI3OutMax=[]  SumI4OutMin=[]  SumI4OutMax=[]  SumDOutMin=[]  SumDOutMax=[]  DifferentiatorOutMin=[]  DifferentiatorOutMax=[]  FilterDiffOutCoefMin=[]  FilterDiffOutCoefMax=[]  ReciprocalOutMin=[]  ReciprocalOutMax=[]  SumDenOutMin=[]  SumDenOutMax=[]  SumNumOutMin=[]  SumNumOutMax=[]  DivideOutMin=[]  DivideOutMax=[]  IntegratorContinuousStateAttributes=''  IntegratorStateMustResolveToSignalObject=off  IntegratorRTWStateStorageClass=Auto  FilterContinuousStateAttributes=''  FilterStateMustResolveToSignalObject=off  FilterRTWStateStorageClass=Auto  ParallelPVariant=InternalParameters  IdealPVariant=Disabled  IVariant=InternalParameters  DVariant=InternalParameters  IntegratorVariant=Continuous  SatVariant=Enabled  AWVariant=ContClampingParallel  PCopyVariant=Disabled  TRVariant=Disabled  FdbkBlocksVariant=Forward  IdealPFdbkVariant=Disabled  SatFdbkVariant=Disabled  DerivativeFilterVariant=ContFilter  NVariant=InternalParameters  NCopyVariant=Disabled  FilterICVariant=InternalICsFilter  IntegratorICVariant=InternalICs  ExternalResetVariant=Disabled  TRSumVariant=Passthrough  SumFdbkVariant=Disabled  SumVariant=Sum_PID
  PID Knee : simulink/Continuous/PID Controller  Controller=PID  Form=Parallel  TimeDomain=Continuous-time  SampleTime=-1  IntegratorMethod=Forward Euler  FilterMethod=Forward Euler  ControllerParametersSource=internal  P=knee_servo_kp  I=knee_servo_ki  D=knee_servo_kd  UseFilter=on  N=deriv_filter_coeff  TunerSelectOption=Transfer Function Based (PID Tuner App)  ZeroCross=off  InitialConditionSource=internal  InitialConditionForIntegrator=0  InitialConditionForFilter=0  DifferentiatorICPrevScaledInput=0  ExternalReset=none  TrackingMode=off  Kt=1  LimitOutput=on  UpperSaturationLimit=max_torque  LowerSaturationLimit=-max_torque  LinearizeAsGain=on  AntiWindupMode=clamping  Kb=1  POutMin=[]  POutMax=[]  IOutMin=[]  IOutMax=[]  DOutMin=[]  DOutMax=[]  NOutMin=[]  NOutMax=[]  SumOutMin=[]  SumOutMax=[]  SaturationOutMin=[]  SaturationOutMax=[]  PParamMin=[]  PParamMax=[]  IParamMin=[]  IParamMax=[]  DParamMin=[]  DParamMax=[]  NParamMin=[]  NParamMax=[]  KbParamMin=[]  KbParamMax=[]  KtParamMin=[]  KtParamMax=[]  KbOutMin=[]  KbOutMax=[]  KtOutMin=[]  KtOutMax=[]  IntegratorOutMin=[]  IntegratorOutMax=[]  FilterOutMin=[]  FilterOutMax=[]  SumI1OutMin=[]  SumI1OutMax=[]  SumI2OutMin=[]  SumI2OutMax=[]  SumI3OutMin=[]  SumI3OutMax=[]  SumI4OutMin=[]  SumI4OutMax=[]  SumDOutMin=[]  SumDOutMax=[]  DifferentiatorOutMin=[]  DifferentiatorOutMax=[]  FilterDiffOutCoefMin=[]  FilterDiffOutCoefMax=[]  ReciprocalOutMin=[]  ReciprocalOutMax=[]  SumDenOutMin=[]  SumDenOutMax=[]  SumNumOutMin=[]  SumNumOutMax=[]  DivideOutMin=[]  DivideOutMax=[]  IntegratorContinuousStateAttributes=''  IntegratorStateMustResolveToSignalObject=off  IntegratorRTWStateStorageClass=Auto  FilterContinuousStateAttributes=''  FilterStateMustResolveToSignalObject=off  FilterRTWStateStorageClass=Auto  ParallelPVariant=InternalParameters  IdealPVariant=Disabled  IVariant=InternalParameters  DVariant=InternalParameters  IntegratorVariant=Continuous  SatVariant=Enabled  AWVariant=ContClampingParallel  PCopyVariant=Disabled  TRVariant=Disabled  FdbkBlocksVariant=Forward  IdealPFdbkVariant=Disabled  SatFdbkVariant=Disabled  DerivativeFilterVariant=ContFilter  NVariant=InternalParameters  NCopyVariant=Disabled  FilterICVariant=InternalICsFilter  IntegratorICVariant=InternalICs  ExternalResetVariant=Disabled  TRSumVariant=Passthrough  SumFdbkVariant=Disabled  SumVariant=Sum_PID
  Sum{1..3,6..8} (6 alike) : Sum  Inputs=|+-
  Input : Outport  VectorParamsAs1DForOutWhenUnconnected=off
  wires:
  Low-Pass Filter5/1 -> Sum8/1
  Low-Pass Filter/1 -> Sum6/1
  Bus Selector4/6 -> Low-Pass Filter5/1  "<hip yaw>"
  PID Hip Roll/1 -> Bus Creator/5  "hip roll"
  Bus Selector4/2 -> Low-Pass Filter1/1  "<ankle pitch>"
  Bus Selector4/4 -> Low-Pass Filter3/1  "<hip pitch>"
  PID Ankle Pitch/1 -> Bus Creator/2  "ankle pitch"
  PID Hip Yaw/1 -> Bus Creator/6  "hip yaw"
  PID Knee/1 -> Bus Creator/3  "knee"
  Bus Selector4/3 -> Low-Pass Filter2/1  "<knee>"
  Bus Selector4/1 -> Low-Pass Filter/1  "<ankle roll>"
  Sum6/1 -> PID Ankle Roll/1
  Bus Selector/3 -> Sum2/2  "<knee_angle>"
  Sum7/1 -> PID Hip Roll/1
  Bus Selector4/5 -> Low-Pass Filter4/1  "<hip roll>"
  Sum3/1 -> PID Hip Pitch/1
  ref/1 -> Bus Selector4/1
  Sum2/1 -> PID Knee/1
  Sum1/1 -> PID Ankle Pitch/1
  PID Ankle Roll/1 -> Bus Creator/1  "ankle roll"
  Low-Pass Filter3/1 -> Sum3/1
  Bus Selector/6 -> Sum8/2  "<hipyaw_angle>"
  PID Hip Pitch/1 -> Bus Creator/4  "hip pitch"
  Bus Selector/5 -> Sum7/2  "<hiproll_angle>"
  Low-Pass Filter1/1 -> Sum1/1
  Bus Creator/1 -> Input/1
  Bus Selector/1 -> Sum6/2  "<ankleroll_angle>"
  Sum8/1 -> PID Hip Yaw/1
  Low-Pass Filter2/1 -> Sum2/1
  Low-Pass Filter4/1 -> Sum7/1
  Bus Selector/4 -> Sum3/2  "<hippitch_angle>"
  Bus Selector/2 -> Sum1/2  "<anklepitch_angle>"
  meas/1 -> Bus Selector/1

== system walkingRobotUtils/Walking Robot (Control Design)/Robot Joint Controller/Motion ==
  refR : Inport
  refL : Inport  Port=2
  measR : Inport  Port=3
  measL : Inport  Port=4
  Terminator : Terminator
  Terminator1 : Terminator
  InputR : Outport  VectorParamsAs1DForOutWhenUnconnected=off
  InputL : Outport  Port=2  VectorParamsAs1DForOutWhenUnconnected=off
  wires:
  refL/1 -> InputL/1
  refR/1 -> InputR/1
  measL/1 -> Terminator/1
  measR/1 -> Terminator1/1

== system walkingRobotUtils/Walking Robot (Control Design)/Robot Joint Controller/Motor ==
  refR : Inport
  measR : Inport  Port=2
  refL : Inport  Port=3
  measL : Inport  Port=4
  PID Controllers L : Subsystem
  PID Controllers R : Subsystem
  InputR : Outport  VectorParamsAs1DForOutWhenUnconnected=off
  InputL : Outport  Port=2  VectorParamsAs1DForOutWhenUnconnected=off
  wires:
  refL/1 -> PID Controllers L/1(ref)
  PID Controllers R/1(Input) -> InputR/1
  measR/1 -> PID Controllers R/2(meas)
  refR/1 -> PID Controllers R/1(ref)
  PID Controllers L/1(Input) -> InputL/1
  measL/1 -> PID Controllers L/2(meas)

== system walkingRobotUtils/Walking Robot (Control Design)/Robot Joint Controller/Torque ==
  refR : Inport
  measR : Inport  Port=2
  refL : Inport  Port=3
  measL : Inport  Port=4
  PID Controllers L : Subsystem
  PID Controllers R : Subsystem
  InputR : Outport  VectorParamsAs1DForOutWhenUnconnected=off
  InputL : Outport  Port=2  VectorParamsAs1DForOutWhenUnconnected=off
  wires:
  measL/1 -> PID Controllers L/2(meas)
  PID Controllers L/1(Input) -> InputL/1
  refR/1 -> PID Controllers R/1(ref)
  measR/1 -> PID Controllers R/2(meas)
  PID Controllers R/1(Input) -> InputR/1
  refL/1 -> PID Controllers L/1(ref)
